simulink model "Modeling_DC_Motor_simulink"  (R2020b)
settings: Solver=VariableStepAuto  StartTime=0.0  StopTime=20  RelTol=1e-3
values from neighbouring files (symbols this model uses):
  B = (650+16.1)*10^-6    (= 0.0006661)    [Modeling_DC_Motor_script.m]
  J = 8*10^-3+57.8*10^-6    (= 0.0080578)    [Modeling_DC_Motor_script.m]
  K_e = 0.094    [Modeling_DC_Motor_script.m]
  K_t = 0.094    [Modeling_DC_Motor_script.m]
  L_a = 528*10^-6    (= 0.000528)    [Modeling_DC_Motor_script.m]
  R_a = 0.649    [Modeling_DC_Motor_script.m]
libraries: simulink x1
settings Model: Creator=rinconm  LastModifiedBy=marco

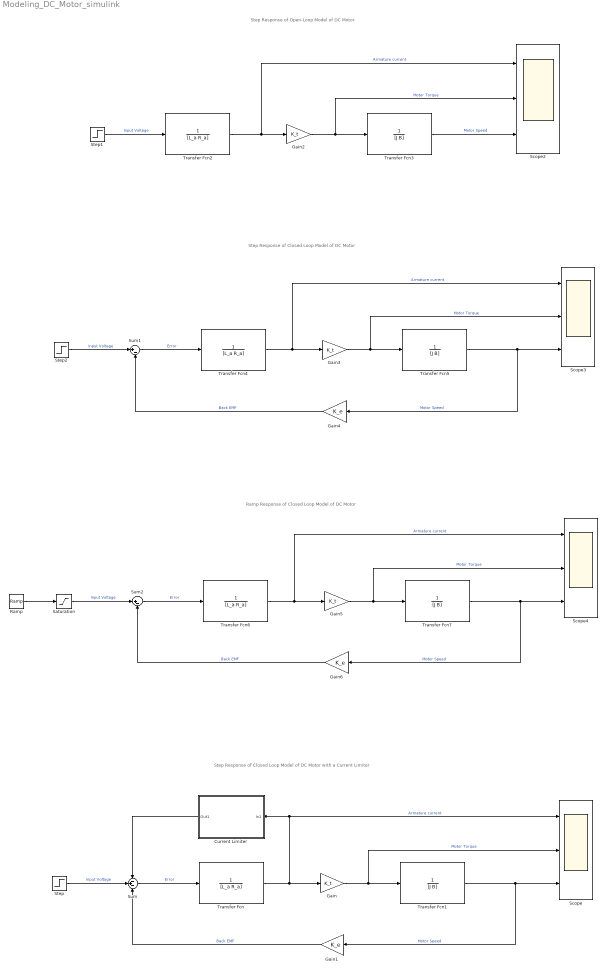
== system Modeling_DC_Motor_simulink ==
  note: Step Response of Closed Loop Model of DC Motor with a Current Limiter
  note: Step Response of Open-Loop Model of DC Motor
  note: Step Response of Closed Loop Model of DC Motor
  note: Ramp Response of Closed Loop Model of DC Motor
  Current Limiter : Subsystem
  Gain{,2..3,5} (4 alike) : Gain  Gain=K_t
  Gain1 : Gain  Gain=K_e
  Gain4 : Gain  Gain=K_e
  Gain6 : Gain  Gain=K_e
  Ramp : simulink/Sources/Ramp  slope=6  start=1  InitialOutput=0
  Saturation : Saturate  UpperLimit=48  LowerLimit=0
  Scope{,2..4} (4 alike) : Scope  NumInputPorts=3
  Step : Step  After=48  SampleTime=0
  Step1 : Step  After=48  SampleTime=0
  Step2 : Step  After=48  SampleTime=0
  Sum : Sum  Inputs=-+-
  Sum1 : Sum  Inputs=|+-
  Sum2 : Sum  Inputs=|+-
  Transfer Fcn{,2,4,6} (4 alike) : TransferFcn  Denominator=[L_a R_a]
  Transfer Fcn{1,3,5,7} (4 alike) : TransferFcn  Denominator=[J B]
  wires:
  Sum/1 -> Transfer Fcn/1  "Error"
  Transfer Fcn/1 -> Current Limiter/1(In1), Scope/1, Gain/1  "Armature current"
  Transfer Fcn1/1 -> Scope/3, Gain1/1  "Motor Speed"
  Gain/1 -> Scope/2, Transfer Fcn1/1  "Motor Torque"
  Step/1 -> Sum/2  "Input Voltage"
  Gain1/1 -> Sum/3  "Back EMF"
  Ramp/1 -> Saturation/1
  Current Limiter/1(Out1) -> Sum/1
  Gain2/1 -> Scope2/2, Transfer Fcn3/1  "Motor Torque"
  Transfer Fcn3/1 -> Scope2/3  "Motor Speed"
  Transfer Fcn2/1 -> Scope2/1, Gain2/1  "Armature current"
  Step1/1 -> Transfer Fcn2/1  "Input Voltage"
  Gain3/1 -> Scope3/2, Transfer Fcn5/1  "Motor Torque"
  Gain4/1 -> Sum1/2  "Back EMF"
  Transfer Fcn5/1 -> Scope3/3, Gain4/1  "Motor Speed"
  Transfer Fcn4/1 -> Scope3/1, Gain3/1  "Armature current"
  Step2/1 -> Sum1/1  "Input Voltage"
  Sum1/1 -> Transfer Fcn4/1  "Error"
  Gain5/1 -> Scope4/2, Transfer Fcn7/1  "Motor Torque"
  Transfer Fcn7/1 -> Scope4/3, Gain6/1  "Motor Speed"
  Saturation/1 -> Sum2/1  "Input Voltage"
  Transfer Fcn6/1 -> Scope4/1, Gain5/1  "Armature current"
  Gain6/1 -> Sum2/2  "Back EMF"
  Sum2/1 -> Transfer Fcn6/1  "Error"

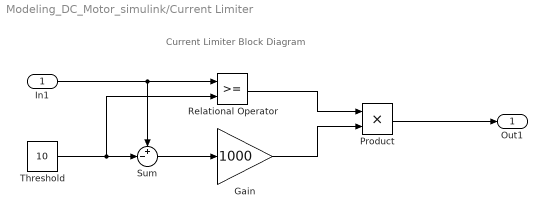
== system Modeling_DC_Motor_simulink/Current Limiter ==
  note: Current Limiter Block Diagram
  In1 : Inport
  Gain : Gain  Gain=1000
  Product : Product
  Relational Operator : RelationalOperator  OutDataTypeStr=boolean  RndMeth=Simplest
  Sum : Sum  Inputs=+-|
  Threshold : Constant  Value=10
  Out1 : Outport
  wires:
  In1/1 -> Sum/1, Relational Operator/1
  Threshold/1 -> Sum/2, Relational Operator/2
  Sum/1 -> Gain/1
  Product/1 -> Out1/1
  Gain/1 -> Product/2
  Relational Operator/1 -> Product/1
